simulink model "podb2012B"  (R2012b)
settings: Solver=ode45  StartTime=0.0  StopTime=500  RelTol=1e-3
undefined symbols (not defined in the file): A1, A2, mi1, mi2, mu1
settings Model: Creator=Sandra Knezevic  LastModifiedBy=Aldin
settings OptimizationCC: ExpressionDepthLimit=128
settings DebuggingCC: UnderspecifiedInitializationDetection=Simplified  MergeDetectMultiDrivingBlocksExec=error  SolverPrmCheckMsg=none  FrameProcessingCompatibilityMsg=error  StateNameClashWarn=none
settings CodeAppCC: CustomSymbolStrType=$N$R$M_T
settings GRTTargetCC: CodeReplacementLibrary=C89/C90 (ANSI)

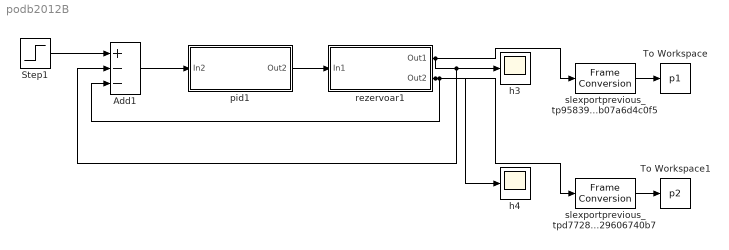
== system podb2012B ==
  Add1 : Sum  Inputs=+--
  Step1 : Step  Time=0  Before=1  After=15  SampleTime=0
  To Workspace : ToWorkspace  VariableName=p1  SampleTime=-1
  To Workspace1 : ToWorkspace  VariableName=p2  SampleTime=-1
  h3 : Scope
      settings: TimeRange=auto  LimitDataPoints=on  MaxDataPoints=5000  SaveToWorkspace=off  SaveName=ScopeData2  YMin=-10  YMax=10  SampleTime=-1  DataFormat=Array
  h4 : Scope
      settings: TimeRange=auto  LimitDataPoints=on  MaxDataPoints=5000  SaveToWorkspace=off  SaveName=ScopeData3  YMin=-10  YMax=10  SampleTime=-1  DataFormat=Array
  pid1 : Subsystem
  rezervoar1 : Subsystem
  slexportprevious_tp95839e7f_5ca1_4183_9947_8b07a6d4c0f5 : FrameConversion  OutFrame=Sample-based
  slexportprevious_tpd7728486_3d1e_4ac9_8066_2529606740b7 : FrameConversion  OutFrame=Sample-based
  wires:
  pid1/1(Out2) -> rezervoar1/1(In1)
  Add1/1 -> pid1/1(In2)
  Step1/1 -> Add1/1
  rezervoar1/1(Out1) -> Add1/2, h3/1, slexportprevious_tp95839e7f_5ca1_4183_9947_8b07a6d4c0f5/1
  rezervoar1/2(Out2) -> Add1/3, h4/1, slexportprevious_tpd7728486_3d1e_4ac9_8066_2529606740b7/1
  slexportprevious_tp95839e7f_5ca1_4183_9947_8b07a6d4c0f5/1 -> To Workspace/1
  slexportprevious_tpd7728486_3d1e_4ac9_8066_2529606740b7/1 -> To Workspace1/1

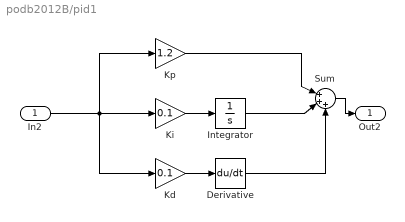
== system podb2012B/pid1 ==
  In2 : Inport
  Derivative : Derivative
  Integrator : Integrator
  Kd : Gain  Gain=0.1
  Ki : Gain  Gain=0.1
  Kp : Gain  Gain=1.2
  Sum : Sum  Inputs=|+++
  Out2 : Outport
  wires:
  Kp/1 -> Sum/1
  Integrator/1 -> Sum/2
  Derivative/1 -> Sum/3
  Sum/1 -> Out2/1
  In2/1 -> Kp/1, Kd/1, Ki/1
  Ki/1 -> Integrator/1
  Kd/1 -> Derivative/1

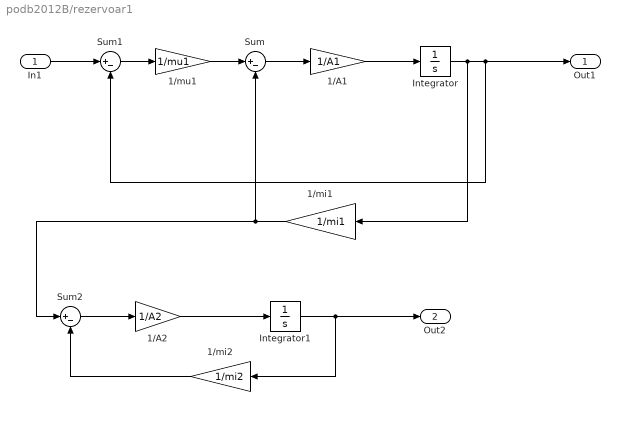
== system podb2012B/rezervoar1 ==
  In1 : Inport
  1/A1 : Gain  Gain=1/A1
  1/A2 : Gain  Gain=1/A2
  1/mi1 : Gain  Gain=1/mi1
  1/mi2 : Gain  Gain=1/mi2
  1/mu1 : Gain  Gain=1/mu1
  Integrator : Integrator  InitialCondition=1
  Integrator1 : Integrator  InitialCondition=1
  Sum : Sum  Inputs=|+-
  Sum1 : Sum  Inputs=|+-
  Sum2 : Sum  Inputs=|+-
  Out1 : Outport
  Out2 : Outport  Port=2
  wires:
  1/A1/1 -> Integrator/1
  1/mu1/1 -> Sum/1
  Sum/1 -> 1/A1/1
  Sum1/1 -> 1/mu1/1
  In1/1 -> Sum1/1
  Integrator/1 -> 1/mi1/1, Sum1/2, Out1/1
  1/mi1/1 -> Sum/2, Sum2/1
  Sum2/1 -> 1/A2/1
  1/A2/1 -> Integrator1/1
  Integrator1/1 -> Out2/1, 1/mi2/1
  1/mi2/1 -> Sum2/2
